simulink library "sm_trackV_lib_chain_underc_i1u2l7"  (R2026a)
settings: Solver=VariableStepAuto
undefined symbols (not defined in the file): Excv, Left, P1, P2, P3, P4, P5, P6, P7, P8, P9, Right
libraries: sm_trackV_lib_chain_underc_elem x26, sm_lib x24, nesl_utility x20, fl_lib x4, sm_trackV_lib_frame_i1u2l7 x2
(part 1 of 2)
Description:
  | Copyright 2023-2026 The MathWorks, Inc.
settings Model: Creator=smiller  LastModifiedBy=smiller

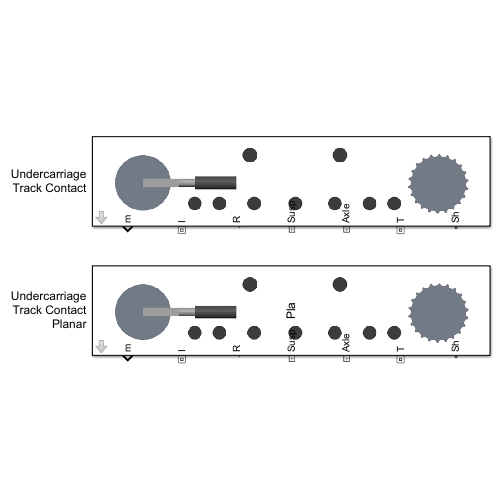
[thumbnail: Simulink's stored preview of the top-level diagram]
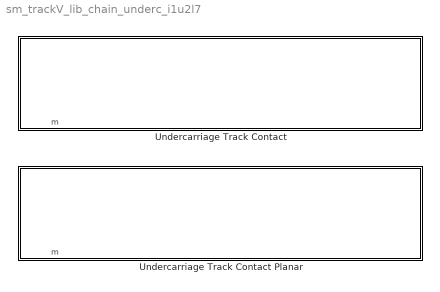
== system sm_trackV_lib_chain_underc_i1u2l7 ==
  Undercarriage Track Contact : Subsystem  mask(Undercarriage for Integration with Track Model){popup_leftOrRight=Left, sprk_xc=Excv.Sprocket.sprocket_xc, sprk_len=Excv.Sprocket.sprk_width, sprk_rho=Excv.Sprocket.density, sprk_clr=Excv.Sprocket.clr, sprk_opc=Excv.Sprocket.opc, sprk_contact_geo_ptcld=Excv.Sprocket.teeth_contact.ptcld.pts, sprk_contact_geo_rad=Excv.Sprocket.teeth_contact.ptcld.rad, sprk_contact_geo_clr=Excv.Sprocket.teeth_contact.ptcld.clr, sprk_contact_geo_opc=Excv.Sprocket.teeth_contact.ptcld.opc, idler_rad=Excv.Idler.rad, idler_len=Excv.Idler.len, idler_rho=Excv.Idler.rho, idler_clr=Excv.Idler.clr, idler_opc=Excv.Idler.opc, idler_contgeo_clr=Excv.Idler.chain_contact.clr, idler_contgeo_opc=Excv.Idler.chain_contact.opc, roller_upper_rad=Excv.Roller.Upper.rad, roller_upper_len=Excv.Roller.Upper.len, roller_upper_rho=Excv.Roller.Upper.rho, roller_upper_clr=Excv.Roller.Upper.clr, roller_upper_opc=Excv.Roller.Upper.opc, roller_upper_contgeo_clr=[1.0 0.0 0.0], roller_upper_contgeo_opc=1, roller_lower_rad=Excv.Roller.Lower.rad, roller_lower_len=Excv.Roller.Lower.len, roller_lower_rho=Excv.Roller.Lower.rho, roller_lower_clr=Excv.Roller.Lower.clr, roller_lower_opc=Excv.Roller.Lower.opc, roller_lower_contgeo_clr=[1.0 0.0 0.0], roller_lower_contgeo_opc=1, tensioner_cyl_len=Excv.Idler.Tensioner.cyl.len, tensioner_cyl_rad=Excv.Idler.Tensioner.cyl.rad, tensioner_cyl_rho=Excv.Idler.Tensioner.cyl.rho, tensioner_cyl_clr=Excv.Idler.Tensioner.cyl.clr, tensioner_cyl_opc=Excv.Idler.Tensioner.cyl.opc, tensioner_pist_len=Excv.Idler.Tensioner.piston.len, tensioner_pist_rad=Excv.Idler.Tensioner.piston.rad, tensioner_pist_rho=Excv.Idler.Tensioner.piston.rho, tensioner_pist_clr=Excv.Idler.Tensioner.piston.clr, tensioner_pist_opc=Excv.Idler.Tensioner.piston.opc, tensioner_br_length=Excv.Idler.Tensioner.bracket.len, tensioner_br_width=Excv.Idler.Tensioner.bracket.wid, tensioner_br_height=Excv.Idler.Tensioner.bracket.height, tensioner_br_thk=Excv.Idler.Tensioner.bracket.thk, tensioner_br_rho=Excv.Idler.Tensioner.bracket.rho, tensioner_br_clr=Excv.Idler.Tensioner.bracket.clr, tensioner_br_opc=Excv.Idler.Tensioner.bracket.opc, tensioner_eqpos=Excv.Idler.Tensioner.xeq, tensioner_x0=Excv.Idler.Tensioner.x0, tensioner_k=Excv.Idler.Tensioner.K, tensioner_b=Excv.Idler.Tensioner.B, roller_upper_x=Excv.Frame.Sprk2UpperX, roller_lower_x=Excv.Frame.Sprk2LowerX, idler_x=Excv.Frame.IdlerAssyX, axle_x=Excv.Frame.AxleX, roller_upper_y=Excv.Frame.Sprk2UpperY, roller_lower_y=Excv.Frame.Sprk2LowerY, idler_y=Excv.Frame.Sprk2IdlerY, axle_y=Excv.Frame.AxleY, frame_cg_offset=Excv.Frame.CGOffset, frame_mass=Excv.Frame.Mass, frame_moi=Excv.Frame.MOI, frame_poi=Excv.Frame.POI, frame_susp_offset=Excv.Frame.SuspOffset, popup_sense_roller=Actuator Torque}
      mask prompts: popup_leftOrRight "Left or Right"; sprk_xc "Extrusion Data [x y] (m)"; sprk_len "Length (m)"; sprk_rho "Density (kg/m^3)"; sprk_clr "Color [R G B] (0-1)"; sprk_opc "Opacity (0-1)"; sprk_contact_geo_ptcld "Point Cloud Data [x y z] (m)"; sprk_contact_geo_rad "Radius (m)"; sprk_contact_geo_clr "Color [R G B] (0-1)"; sprk_contact_geo_opc "Opacity (0-1)"; idler_rad "Radius (m)"; idler_len "Length (m)"; idler_rho "Density (kg/m^3)"; idler_clr "Color [R G B] (0-1)"; idler_opc "Opacity (0-1)"; idler_contgeo_clr "Color [R G B] (0-1)"; idler_contgeo_opc "Opacity (0-1)"; roller_upper_rad "Radius (m)"; roller_upper_len "Length (m)"; roller_upper_rho "Density (kg/m^3)"; roller_upper_clr "Color [R G B] (0-1)"; roller_upper_opc "Opacity (0-1)"; roller_upper_contgeo_clr "Color [R G B] (0-1)"; roller_upper_contgeo_opc "Opacity (0-1)"; roller_lower_rad "Radius (m)"; roller_lower_len "Length (m)"; roller_lower_rho "Density (kg/m^3)"; roller_lower_clr "Color [R G B] (0-1)"; roller_lower_opc "Opacity (0-1)"; roller_lower_contgeo_clr "Color [R G B] (0-1)"; roller_lower_contgeo_opc "Opacity (0-1)"; tensioner_cyl_len "Length (m)"; tensioner_cyl_rad "Radius (m)"; tensioner_cyl_rho "Density (kg/m^3)"; tensioner_cyl_clr "Color [R G B] (0-1)"; tensioner_cyl_opc "Opacity (0-1)"; tensioner_pist_len "Length (m)"; tensioner_pist_rad "Radius (m)"; tensioner_pist_rho "Density (kg/m^3)"; tensioner_pist_clr "Color [R G B] (0-1)"; tensioner_pist_opc "Opacity (0.1)"; tensioner_br_length "Length (m)"; tensioner_br_width "Width (m)"; tensioner_br_height "Height (m)"; tensioner_br_thk "Thickness (m)"; tensioner_br_rho "Density (kg/m^3)"; tensioner_br_clr "Color [R G B] (0-1)"; tensioner_br_opc "Opacity (0.1)"; tensioner_eqpos "Equilibrium Position (m)"; tensioner_x0 "Assembly Position (m)"; tensioner_k "Stiffness Coefficient (N/m)"; tensioner_b "Damping Coefficient (N/(m/s))"; roller_upper_x "Upper Rollers (vector) (m)"; roller_lower_x "Lower Rollers (vector) (m)"; idler_x "Idler Wheel (m)"; axle_x "Axle (m)"; roller_upper_y "Sprocket to Upper Rollers (m)"; roller_lower_y "Sprocket to Lower Rollers (m)"; idler_y "Sprocket to Idler (m)"; axle_y "Axle (m)"; frame_cg_offset "CG Offset from Sprocket [x y z] (m)"; frame_mass "Mass (kg)"; frame_moi "Moments of Inertia [Ixx Iyy Izz] (kg*m^2)"; frame_poi "Products of Inertia [Ixx Iyy Izz] (kg*m^2)"; frame_susp_offset "Suspension Offset from Sprocket [x y z] (m)"; popup_sense_roller "Roller"
      mask help: Models sprocket, rollers, and idler with tensioner. Components have contact geometry for integration with a segmented track model. The sprocket has a 1D rotational mechanical interface to the drivetrain.
      mask init:
      | bh = gcb;
      | set_param([bh '/Rollers'],'popup_sense_roller',get_param(bh,'popup_sense_roller'));
      mask TypeOptions popup_leftOrRight: Frame/popup_leftOrRight
      mask TypeOptions sprk_xc: Rollers/sprk_xc
      mask TypeOptions sprk_len: Rollers/sprk_len
      mask TypeOptions sprk_rho: Rollers/sprk_rho
      mask TypeOptions sprk_clr: Rollers/sprk_clr
      mask TypeOptions sprk_opc: Rollers/sprk_opc
      mask TypeOptions sprk_contact_geo_ptcld: Rollers/sprk_contact_geo_ptcld
      mask TypeOptions sprk_contact_geo_rad: Rollers/sprk_contact_geo_rad
      mask TypeOptions sprk_contact_geo_clr: Rollers/sprk_contact_geo_clr
      mask TypeOptions sprk_contact_geo_opc: Rollers/sprk_contact_geo_opc
      mask TypeOptions idler_rad: Rollers/idler_rad
      mask TypeOptions idler_len: Rollers/idler_len
      mask TypeOptions idler_rho: Rollers/idler_rho
      mask TypeOptions idler_clr: Rollers/idler_clr
      mask TypeOptions idler_opc: Rollers/idler_opc
      mask TypeOptions idler_contgeo_clr: Rollers/idler_contgeo_clr
      mask TypeOptions idler_contgeo_opc: Rollers/idler_contgeo_opc
      mask TypeOptions roller_upper_rad: Rollers/roller_upper_rad
      mask TypeOptions roller_upper_len: Rollers/roller_upper_len
      mask TypeOptions roller_upper_rho: Rollers/roller_upper_rho
      mask TypeOptions roller_upper_clr: Rollers/roller_upper_clr
      mask TypeOptions roller_upper_opc: Rollers/roller_upper_opc
      mask TypeOptions roller_upper_contgeo_clr: Rollers/roller_upper_contgeo_clr
      mask TypeOptions roller_upper_contgeo_opc: Rollers/roller_upper_contgeo_opc
      mask TypeOptions roller_lower_rad: Rollers/roller_lower_rad
      mask TypeOptions roller_lower_len: Rollers/roller_lower_len
      mask TypeOptions roller_lower_rho: Rollers/roller_lower_rho
      mask TypeOptions roller_lower_clr: Rollers/roller_lower_clr
      mask TypeOptions roller_lower_opc: Rollers/roller_lower_opc
      mask TypeOptions roller_lower_contgeo_clr: Rollers/roller_lower_contgeo_clr
      mask TypeOptions roller_lower_contgeo_opc: Rollers/roller_lower_contgeo_opc
      mask TypeOptions tensioner_cyl_len: Rollers/tensioner_cyl_len
      mask TypeOptions tensioner_cyl_rad: Rollers/tensioner_cyl_rad
      mask TypeOptions tensioner_cyl_rho: Rollers/tensioner_cyl_rho
      mask TypeOptions tensioner_cyl_clr: Rollers/tensioner_cyl_clr
      mask TypeOptions tensioner_cyl_opc: Rollers/tensioner_cyl_opc
      mask TypeOptions tensioner_pist_len: Rollers/tensioner_pist_len
      mask TypeOptions tensioner_pist_rad: Rollers/tensioner_pist_rad
      mask TypeOptions tensioner_pist_rho: Rollers/tensioner_pist_rho
      mask TypeOptions tensioner_pist_clr: Rollers/tensioner_pist_clr
      mask TypeOptions tensioner_pist_opc: Rollers/tensioner_pist_opc
      mask TypeOptions tensioner_br_length: Rollers/tensioner_br_length
      mask TypeOptions tensioner_br_width: Rollers/tensioner_br_width
      mask TypeOptions tensioner_br_height: Rollers/tensioner_br_height
      mask TypeOptions tensioner_br_thk: Rollers/tensioner_br_thk
      mask TypeOptions tensioner_br_rho: Rollers/tensioner_br_rho
      mask TypeOptions tensioner_br_clr: Rollers/tensioner_br_clr
      mask TypeOptions tensioner_br_opc: Rollers/tensioner_br_opc
      mask TypeOptions tensioner_eqpos: Rollers/tensioner_eqpos
      mask TypeOptions tensioner_x0: Rollers/tensioner_x0
      mask TypeOptions tensioner_k: Rollers/tensioner_k
      mask TypeOptions tensioner_b: Rollers/tensioner_b
      mask TypeOptions roller_upper_x: Frame/roller_upper_x
      mask TypeOptions roller_lower_x: Frame/roller_lower_x
      mask TypeOptions idler_x: Frame/idler_x
      mask TypeOptions axle_x: Frame/axle_x
      mask TypeOptions roller_upper_y: Frame/roller_upper_y
      mask TypeOptions roller_lower_y: Frame/roller_lower_y
      mask TypeOptions idler_y: Frame/idler_y
      mask TypeOptions axle_y: Frame/axle_y
      mask TypeOptions frame_cg_offset: Frame/frame_cg_offset
      mask TypeOptions frame_mass: Frame/frame_mass
      mask TypeOptions frame_moi: Frame/frame_moi
      mask TypeOptions frame_poi: Frame/frame_poi
      mask TypeOptions frame_susp_offset: Frame/frame_susp_offset
      mask TypeOptions popup_sense_roller: Constraint Force | Actuator Torque
      mask DialogControl cont_sprocket Prompt: Sprocket
      mask DialogControl cont_sprocket_solid Prompt: Solid
      mask DialogControl cont_sprocket_contact_geo Prompt: Contact Geometry
      mask DialogControl cont_idler Prompt: Idler
      mask DialogControl cont_idler_solid Prompt: Solid
      mask DialogControl cont_idler_contact_geo Prompt: Contact Geometry
      mask DialogControl cont_rollers Prompt: Rollers
      mask DialogControl cont_roller_upper Prompt: Upper
      mask DialogControl cont_roller_upper_contact_geo Prompt: Contact Geometry
      mask DialogControl cont_rollers_lower Prompt: Lower
      mask DialogControl cont_rollers_lower_contact_geo Prompt: Contact Geometry
      mask DialogControl cont_tensioner Prompt: Tensioner
      mask DialogControl cont_tensioner_cyl Prompt: Cylinder
      mask DialogControl cont_tensioner_pist Prompt: Piston
      mask DialogControl cont_tensioner_brkt Prompt: Bracket
      mask DialogControl cont_tensioner_assembly Prompt: Assembly
      mask DialogControl cont_frame Prompt: Frame
      mask DialogControl cont_offset_x Prompt: Longitudinal Offsets from Sprocket
      mask DialogControl cont_offset_y Prompt: Vertical Offsets
      mask DialogControl cont_mass Prompt: Mass and Inertia
      mask DialogControl cont_susp Prompt: Suspension Offsets
      mask DialogControl cont_sensing Prompt: Sensing
      mask Display: image('sm_excv_track_rollers_IMAGE.png');
  Undercarriage Track Contact Planar : Subsystem  mask(Undercarriage for Integration with Track Model){popup_leftOrRight=Right, sprk_xc=Excv.Sprocket.sprocket_xc, sprk_len=Excv.Sprocket.sprk_width, sprk_rho=Excv.Sprocket.density, sprk_clr=Excv.Sprocket.clr, sprk_opc=Excv.Sprocket.opc, sprk_contact_geo_ptcld=Excv.Sprocket.teeth_contact.ptcld.pts, sprk_contact_geo_rad=Excv.Sprocket.teeth_contact.ptcld.rad, sprk_contact_geo_clr=Excv.Sprocket.teeth_contact.ptcld.clr, sprk_contact_geo_opc=Excv.Sprocket.teeth_contact.ptcld.opc, idler_rad=Excv.Idler.rad, idler_len=Excv.Idler.len, idler_rho=Excv.Idler.rho, idler_clr=Excv.Idler.clr, idler_opc=Excv.Idler.opc, idler_contgeo_clr=Excv.Idler.chain_contact.clr, idler_contgeo_opc=Excv.Idler.chain_contact.opc, roller_upper_rad=Excv.Roller.Upper.rad, roller_upper_len=Excv.Roller.Upper.len, roller_upper_rho=Excv.Roller.Upper.rho, roller_upper_clr=Excv.Roller.Upper.clr, roller_upper_opc=Excv.Roller.Upper.opc, roller_upper_contgeo_clr=[1.0 0.0 0.0], roller_upper_contgeo_opc=1, roller_lower_rad=Excv.Roller.Lower.rad, roller_lower_len=Excv.Roller.Lower.len, roller_lower_rho=Excv.Roller.Lower.rho, roller_lower_clr=Excv.Roller.Lower.clr, roller_lower_opc=Excv.Roller.Lower.opc, roller_lower_contgeo_clr=[1.0 0.0 0.0], roller_lower_contgeo_opc=1, tensioner_cyl_len=Excv.Idler.Tensioner.cyl.len, tensioner_cyl_rad=Excv.Idler.Tensioner.cyl.rad, tensioner_cyl_rho=Excv.Idler.Tensioner.cyl.rho, tensioner_cyl_clr=Excv.Idler.Tensioner.cyl.clr, tensioner_cyl_opc=Excv.Idler.Tensioner.cyl.opc, tensioner_pist_len=Excv.Idler.Tensioner.piston.len, tensioner_pist_rad=Excv.Idler.Tensioner.piston.rad, tensioner_pist_rho=Excv.Idler.Tensioner.piston.rho, tensioner_pist_clr=Excv.Idler.Tensioner.piston.clr, tensioner_pist_opc=Excv.Idler.Tensioner.piston.opc, tensioner_br_length=Excv.Idler.Tensioner.bracket.len, tensioner_br_width=Excv.Idler.Tensioner.bracket.wid, tensioner_br_height=Excv.Idler.Tensioner.bracket.height, tensioner_br_thk=Excv.Idler.Tensioner.bracket.thk, tensioner_br_rho=Excv.Idler.Tensioner.bracket.rho, tensioner_br_clr=Excv.Idler.Tensioner.bracket.clr, tensioner_br_opc=Excv.Idler.Tensioner.bracket.opc, tensioner_eqpos=Excv.Idler.Tensioner.xeq, tensioner_x0=Excv.Idler.Tensioner.x0, tensioner_k=Excv.Idler.Tensioner.K, tensioner_b=Excv.Idler.Tensioner.B, roller_upper_x=Excv.Frame.Sprk2UpperX, roller_lower_x=Excv.Frame.Sprk2LowerX, idler_x=Excv.Frame.IdlerAssyX, axle_x=Excv.Frame.AxleX, roller_upper_y=Excv.Frame.Sprk2UpperY, roller_lower_y=Excv.Frame.Sprk2LowerY, idler_y=Excv.Frame.Sprk2IdlerY, axle_y=Excv.Frame.AxleY, frame_cg_offset=Excv.Frame.CGOffset, frame_mass=Excv.Frame.Mass, frame_moi=Excv.Frame.MOI, frame_poi=Excv.Frame.POI, frame_susp_offset=Excv.Frame.SuspOffset, popup_sense_roller=Actuator Torque}
      mask prompts: popup_leftOrRight "Left or Right"; sprk_xc "Extrusion Data [x y] (m)"; sprk_len "Length (m)"; sprk_rho "Density (kg/m^3)"; sprk_clr "Color [R G B] (0-1)"; sprk_opc "Opacity (0-1)"; sprk_contact_geo_ptcld "Point Cloud Data [x y z] (m)"; sprk_contact_geo_rad "Radius (m)"; sprk_contact_geo_clr "Color [R G B] (0-1)"; sprk_contact_geo_opc "Opacity (0-1)"; idler_rad "Radius (m)"; idler_len "Length (m)"; idler_rho "Density (kg/m^3)"; idler_clr "Color [R G B] (0-1)"; idler_opc "Opacity (0-1)"; idler_contgeo_clr "Color [R G B] (0-1)"; idler_contgeo_opc "Opacity (0-1)"; roller_upper_rad "Radius (m)"; roller_upper_len "Length (m)"; roller_upper_rho "Density (kg/m^3)"; roller_upper_clr "Color [R G B] (0-1)"; roller_upper_opc "Opacity (0-1)"; roller_upper_contgeo_clr "Color [R G B] (0-1)"; roller_upper_contgeo_opc "Opacity (0-1)"; roller_lower_rad "Radius (m)"; roller_lower_len "Length (m)"; roller_lower_rho "Density (kg/m^3)"; roller_lower_clr "Color [R G B] (0-1)"; roller_lower_opc "Opacity (0-1)"; roller_lower_contgeo_clr "Color [R G B] (0-1)"; roller_lower_contgeo_opc "Opacity (0-1)"; tensioner_cyl_len "Length (m)"; tensioner_cyl_rad "Radius (m)"; tensioner_cyl_rho "Density (kg/m^3)"; tensioner_cyl_clr "Color [R G B] (0-1)"; tensioner_cyl_opc "Opacity (0-1)"; tensioner_pist_len "Length (m)"; tensioner_pist_rad "Radius (m)"; tensioner_pist_rho "Density (kg/m^3)"; tensioner_pist_clr "Color [R G B] (0-1)"; tensioner_pist_opc "Opacity (0.1)"; tensioner_br_length "Length (m)"; tensioner_br_width "Width (m)"; tensioner_br_height "Height (m)"; tensioner_br_thk "Thickness (m)"; tensioner_br_rho "Density (kg/m^3)"; tensioner_br_clr "Color [R G B] (0-1)"; tensioner_br_opc "Opacity (0.1)"; tensioner_eqpos "Equilibrium Position (m)"; tensioner_x0 "Assembly Position (m)"; tensioner_k "Stiffness Coefficient (N/m)"; tensioner_b "Damping Coefficient (N/(m/s))"; roller_upper_x "Upper Rollers (vector) (m)"; roller_lower_x "Lower Rollers (vector) (m)"; idler_x "Idler Wheel (m)"; axle_x "Axle (m)"; roller_upper_y "Sprocket to Upper Rollers (m)"; roller_lower_y "Sprocket to Lower Rollers (m)"; idler_y "Sprocket to Idler (m)"; axle_y "Sprocket to Axle (m)"; frame_cg_offset "CG Offset from Sprocket [x y z] (m)"; frame_mass "Mass (kg)"; frame_moi "Moments of Inertia [Ixx Iyy Izz] (kg*m^2)"; frame_poi "Products of Inertia [Ixx Iyy Izz] (kg*m^2)"; frame_susp_offset "Suspension Offset from Sprocket [x y z] (m)"; popup_sense_roller "Roller"
      mask help: Models sprocket, rollers, and idler with tensioner. Components have contact geometry for integration with a segmented track model. Contact forces within the track are planar to speed up simulation. The sprocket has a 1D rotational mechanical interface to the drivetrain.
      mask init:
      | bh = gcb;
      | set_param([bh '/Rollers'],'popup_sense_roller',get_param(bh,'popup_sense_roller'));
      mask TypeOptions popup_leftOrRight: Frame/popup_leftOrRight
      mask TypeOptions sprk_xc: Rollers/sprk_xc
      mask TypeOptions sprk_len: Rollers/sprk_len
      mask TypeOptions sprk_rho: Rollers/sprk_rho
      mask TypeOptions sprk_clr: Rollers/sprk_clr
      mask TypeOptions sprk_opc: Rollers/sprk_opc
      mask TypeOptions sprk_contact_geo_ptcld: Rollers/sprk_contact_geo_ptcld
      mask TypeOptions sprk_contact_geo_rad: Rollers/sprk_contact_geo_rad
      mask TypeOptions sprk_contact_geo_clr: Rollers/sprk_contact_geo_clr
      mask TypeOptions sprk_contact_geo_opc: Rollers/sprk_contact_geo_opc
      mask TypeOptions idler_rad: Rollers/idler_rad
      mask TypeOptions idler_len: Rollers/idler_len
      mask TypeOptions idler_rho: Rollers/idler_rho
      mask TypeOptions idler_clr: Rollers/idler_clr
      mask TypeOptions idler_opc: Rollers/idler_opc
      mask TypeOptions idler_contgeo_clr: Rollers/idler_contgeo_clr
      mask TypeOptions idler_contgeo_opc: Rollers/idler_contgeo_opc
      mask TypeOptions roller_upper_rad: Rollers/roller_upper_rad
      mask TypeOptions roller_upper_len: Rollers/roller_upper_len
      mask TypeOptions roller_upper_rho: Rollers/roller_upper_rho
      mask TypeOptions roller_upper_clr: Rollers/roller_upper_clr
      mask TypeOptions roller_upper_opc: Rollers/roller_upper_opc
      mask TypeOptions roller_upper_contgeo_clr: Rollers/roller_upper_contgeo_clr
      mask TypeOptions roller_upper_contgeo_opc: Rollers/roller_upper_contgeo_opc
      mask TypeOptions roller_lower_rad: Rollers/roller_lower_rad
      mask TypeOptions roller_lower_len: Rollers/roller_lower_len
      mask TypeOptions roller_lower_rho: Rollers/roller_lower_rho
      mask TypeOptions roller_lower_clr: Rollers/roller_lower_clr
      mask TypeOptions roller_lower_opc: Rollers/roller_lower_opc
      mask TypeOptions roller_lower_contgeo_clr: Rollers/roller_lower_contgeo_clr
      mask TypeOptions roller_lower_contgeo_opc: Rollers/roller_lower_contgeo_opc
      mask TypeOptions tensioner_cyl_len: Rollers/tensioner_cyl_len
      mask TypeOptions tensioner_cyl_rad: Rollers/tensioner_cyl_rad
      mask TypeOptions tensioner_cyl_rho: Rollers/tensioner_cyl_rho
      mask TypeOptions tensioner_cyl_clr: Rollers/tensioner_cyl_clr
      mask TypeOptions tensioner_cyl_opc: Rollers/tensioner_cyl_opc
      mask TypeOptions tensioner_pist_len: Rollers/tensioner_pist_len
      mask TypeOptions tensioner_pist_rad: Rollers/tensioner_pist_rad
      mask TypeOptions tensioner_pist_rho: Rollers/tensioner_pist_rho
      mask TypeOptions tensioner_pist_clr: Rollers/tensioner_pist_clr
      mask TypeOptions tensioner_pist_opc: Rollers/tensioner_pist_opc
      mask TypeOptions tensioner_br_length: Rollers/tensioner_br_length
      mask TypeOptions tensioner_br_width: Rollers/tensioner_br_width
      mask TypeOptions tensioner_br_height: Rollers/tensioner_br_height
      mask TypeOptions tensioner_br_thk: Rollers/tensioner_br_thk
      mask TypeOptions tensioner_br_rho: Rollers/tensioner_br_rho
      mask TypeOptions tensioner_br_clr: Rollers/tensioner_br_clr
      mask TypeOptions tensioner_br_opc: Rollers/tensioner_br_opc
      mask TypeOptions tensioner_eqpos: Rollers/tensioner_eqpos
      mask TypeOptions tensioner_x0: Rollers/tensioner_x0
      mask TypeOptions tensioner_k: Rollers/tensioner_k
      mask TypeOptions tensioner_b: Rollers/tensioner_b
      mask TypeOptions roller_upper_x: Frame/roller_upper_x
      mask TypeOptions roller_lower_x: Frame/roller_lower_x
      mask TypeOptions idler_x: Frame/idler_x
      mask TypeOptions axle_x: Frame/axle_x
      mask TypeOptions roller_upper_y: Frame/roller_upper_y
      mask TypeOptions roller_lower_y: Frame/roller_lower_y
      mask TypeOptions idler_y: Frame/idler_y
      mask TypeOptions axle_y: Frame/axle_y
      mask TypeOptions frame_cg_offset: Frame/frame_cg_offset
      mask TypeOptions frame_mass: Frame/frame_mass
      mask TypeOptions frame_moi: Frame/frame_moi
      mask TypeOptions frame_poi: Frame/frame_poi
      mask TypeOptions frame_susp_offset: Frame/frame_susp_offset
      mask TypeOptions popup_sense_roller: Constraint Force | Actuator Torque
      mask DialogControl cont_sprocket Prompt: Sprocket
      mask DialogControl cont_sprocket_solid Prompt: Solid
      mask DialogControl cont_sprocket_contact_geo Prompt: Contact Geometry
      mask DialogControl cont_idler Prompt: Idler
      mask DialogControl cont_idler_solid Prompt: Solid
      mask DialogControl cont_idler_contact_geo Prompt: Contact Geometry
      mask DialogControl cont_rollers Prompt: Rollers
      mask DialogControl cont_roller_upper Prompt: Upper
      mask DialogControl cont_roller_upper_contact_geo Prompt: Contact Geometry
      mask DialogControl cont_rollers_lower Prompt: Lower
      mask DialogControl cont_rollers_lower_contact_geo Prompt: Contact Geometry
      mask DialogControl cont_tensioner Prompt: Tensioner
      mask DialogControl cont_tensioner_cyl Prompt: Cylinder
      mask DialogControl cont_tensioner_pist Prompt: Piston
      mask DialogControl cont_tensioner_brkt Prompt: Bracket
      mask DialogControl cont_tensioner_assembly Prompt: Assembly
      mask DialogControl cont_frame Prompt: Frame
      mask DialogControl cont_offset_x Prompt: Longitudinal Offsets from Sprocket
      mask DialogControl cont_offset_y Prompt: Vertical Offsets
      mask DialogControl cont_mass Prompt: Mass and Inertia
      mask DialogControl cont_susp Prompt: Suspension Offset
      mask DialogControl cont_sensing Prompt: Sensing
      mask Display:
      | image('sm_excv_track_rollers_IMAGE.png');
      | disp('Pla');

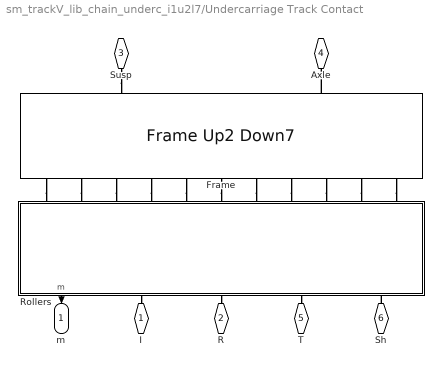
== system sm_trackV_lib_chain_underc_i1u2l7/Undercarriage Track Contact ==
  Frame : sm_trackV_lib_frame_i1u2l7/Frame Up2 Down7  popup_leftOrRight=Left  roller_upper_x=roller_upper_x  roller_lower_x=roller_lower_x  idler_x=idler_x  axle_x=axle_x  roller_upper_y=roller_upper_y  roller_lower_y=roller_lower_y  idler_y=idler_y  axle_y=axle_y  frame_cg_offset=frame_cg_offset  frame_mass=frame_mass  frame_moi=frame_moi  frame_poi=frame_poi  frame_susp_offset=frame_susp_offset
  Rollers : Subsystem  mask(Rollers for Integration with Track Model){sprk_xc=sprk_xc, sprk_len=sprk_len, sprk_rho=sprk_rho, sprk_clr=sprk_clr, sprk_opc=sprk_opc, sprk_contact_geo_ptcld=sprk_contact_geo_ptcld, sprk_contact_geo_rad=sprk_contact_geo_rad, sprk_contact_geo_clr=sprk_contact_geo_clr, sprk_contact_geo_opc=sprk_contact_geo_opc, idler_rad=idler_rad, idler_len=idler_len, idler_rho=idler_rho, idler_clr=idler_clr, idler_opc=idler_opc, idler_contgeo_clr=idler_contgeo_clr, idler_contgeo_opc=idler_contgeo_opc, roller_upper_len=roller_upper_len, roller_upper_rad=roller_upper_rad, roller_upper_rho=roller_upper_rho, roller_upper_clr=roller_upper_clr, roller_upper_opc=roller_upper_opc, roller_upper_contgeo_clr=roller_upper_contgeo_clr, roller_upper_contgeo_opc=roller_upper_contgeo_opc, roller_lower_len=roller_lower_len, roller_lower_rad=roller_lower_rad, roller_lower_rho=roller_lower_rho, roller_lower_clr=roller_lower_clr, roller_lower_opc=roller_lower_opc, roller_lower_contgeo_clr=roller_lower_contgeo_clr, roller_lower_contgeo_opc=roller_lower_contgeo_opc, tensioner_cyl_rad=tensioner_cyl_rad, tensioner_cyl_len=tensioner_cyl_len, tensioner_cyl_rho=tensioner_cyl_rho, tensioner_cyl_clr=tensioner_cyl_clr, tensioner_cyl_opc=tensioner_cyl_opc, tensioner_pist_rad=tensioner_pist_rad, tensioner_pist_len=tensioner_pist_len, tensioner_pist_rho=tensioner_pist_rho, tensioner_pist_clr=tensioner_pist_clr, tensioner_pist_opc=tensioner_pist_opc, tensioner_br_length=tensioner_br_length, tensioner_br_width=tensioner_br_width, tensioner_br_height=tensioner_br_height, tensioner_br_thk=tensioner_br_thk, tensioner_br_rho=tensioner_br_rho, tensioner_br_clr=tensioner_br_clr, tensioner_br_opc=tensioner_br_opc, tensioner_eqpos=tensioner_eqpos, tensioner_x0=tensioner_x0, tensioner_b=tensioner_b, tensioner_k=tensioner_k, popup_sense_roller=Actuator Torque}
      mask prompts: sprk_xc "Extrusion Data [x y] (m)"; sprk_len "Length (m)"; sprk_rho "Density (kg/m^3)"; sprk_clr "Color [R G B] (0-1)"; sprk_opc "Opacity (0-1)"; sprk_contact_geo_ptcld "Point Cloud Data [x y z] (m)"; sprk_contact_geo_rad "Radius (m)"; sprk_contact_geo_clr "Color [R G B] (0-1)"; sprk_contact_geo_opc "Opacity (0-1)"; idler_rad "Radius (m)"; idler_len "Length(m)"; idler_rho "Density (kg/m^3)"; idler_clr "Color [R G B] (0-1)"; idler_opc "Opacity (0-1)"; idler_contgeo_clr "Color [R G B] (0-1)"; idler_contgeo_opc "Opacity (0-1)"; roller_upper_len "Length (m)"; roller_upper_rad "Radius (m)"; roller_upper_rho "Density (kg/m^3)"; roller_upper_clr "Color [R G B] (0-1)"; roller_upper_opc "Opacity (0-1)"; roller_upper_contgeo_clr "Color [R G B] (0-1)"; roller_upper_contgeo_opc "Opacity (0-1)"; roller_lower_len "Length (m)"; roller_lower_rad "Radius (m)"; roller_lower_rho "Density (kg/m^3)"; roller_lower_clr "Color [R G B] (0-1)"; roller_lower_opc "Opacity (0-1)"; roller_lower_contgeo_clr "Color [R G B] (0-1)"; roller_lower_contgeo_opc "Opacity (0-1)"; tensioner_cyl_rad "Radius (m)"; tensioner_cyl_len "Length (m)"; tensioner_cyl_rho "Density (kg/m^3)"; tensioner_cyl_clr "Color [R G B] (0-1)"; tensioner_cyl_opc "Opacity (0-1)"; tensioner_pist_rad "Radius (m)"; tensioner_pist_len "Length (m)"; tensioner_pist_rho "Density (kg/m^3)"; tensioner_pist_clr "Color [R G B] (0-1)"; tensioner_pist_opc "Opacity (0.1)"; tensioner_br_length "Length (m)"; tensioner_br_width "Width (m)"; tensioner_br_height "Height (m)"; tensioner_br_thk "Thickness (m)"; tensioner_br_rho "Density (kg/m^3)"; tensioner_br_clr "Color [R G B] (0-1)"; tensioner_br_opc "Opacity (0.1)"; tensioner_eqpos "Equilibrium Position (m)"; tensioner_x0 "Assembly Position (m)"; tensioner_b "Damping Coefficient (N/(m/s))"; tensioner_k "Stiffness Coefficient (N/m)"; popup_sense_roller "Roller"
      mask help: Models sprocket, rollers, and idler with tensioner. Components have contact geometry for integration with a segmented track model. The sprocket has a 1D rotational mechanical interface to the drivetrain.
      mask init:
      | % Sensing a constraint force can be computationally expensive
      | % Use popup to turn it off if quantity is not needed
      | bh = gcb;
      | if(strcmp(get_param(bh,'popup_sense_roller'),'Constraint Force'))
      |     SCF = 'on'; STF = 'off';
      |     connectedPort = "fc_out";
      |     senseConstraintTorque = "on";
      |     senseTorqueForce = "off";
      | 
      | else
      |     SCF = 'off'; STF = 'on';
      |     connectedPort = "t_out";
      |     senseConstraintTorque = "off";
      |     senseTorqueForce = "on";
      | end
      | 
      | f = Simulink.FindOptions('RegExp',true,'SearchDepth',1);
      | bh_rv = Simulink.findBlocks(bh,'Name','Revolute Lower #*',f);
      | bh_ps = Simulink.findBlocks(bh,'Name','PS-SL Lower #*',f);
      | [~, indrv] = sort(getfullname(bh_rv));
      | [~, indps] = sort(getfullname(bh_ps));
      | bh_rv = bh_rv(indrv);
      | bh_ps = bh_ps(indps);
      | 
      | bh_rvspr = get_param([bh '/Revolute Sprocket'],'Handle');
      | bh_rvidl = get_param([bh '/Revolute Idler'],'Handle');
      | 
      | bh_psspr = get_param([bh '/PS-SL Sprocket'],'Handle');
      | bh_psidl = get_param([bh '/PS-SL Idler'],'Handle');
      | 
      | bh_rv = [bh_rv; bh_rvidl; bh_rvspr];
      | bh_ps = [bh_ps; bh_psidl; bh_psspr];
      | 
      | for i = 1:length(bh_rv)
      |     port_rv = get_param(bh_rv(i),'PortHandles');
      |     port_ps = get_param(bh_ps(i),'PortHandles');
      |     line_rv = get_param(bh_rv(i),'LineHandles');
      | 
      |     if (i==length(bh_rv))
      |         lineInd = 3; % Sprocket joint senses 2 signals
      |     else
      |         lineInd = 2; % All other joints sense 1 signal
      |     end
      |     delete_line(line_rv.RConn(lineInd))
      | 
      |     set_param(bh_rv(i),'SenseConstraintForce',SCF,'SenseTorqueForce',STF);
      |     simscape.addConnection(bh_rv(i), connectedPort, bh_ps(i),'input');
      | 
      | end
      mask TypeOptions sprk_xc: Sprocket/sprk_xc
      mask TypeOptions sprk_len: Sprocket/sprk_len
      mask TypeOptions sprk_rho: Sprocket/sprk_rho
      mask TypeOptions sprk_clr: Sprocket/sprk_clr
      mask TypeOptions sprk_opc: Sprocket/sprk_opc
      mask TypeOptions sprk_contact_geo_ptcld: Sprocket/sprk_contact_geo_ptcld
      mask TypeOptions sprk_contact_geo_rad: Sprocket/sprk_contact_geo_rad
      mask TypeOptions sprk_contact_geo_clr: Sprocket/sprk_contact_geo_clr
      mask TypeOptions sprk_contact_geo_opc: Sprocket/sprk_contact_geo_opc
      mask TypeOptions idler_rad: Idler/idler_rad
      mask TypeOptions idler_len: Idler/idler_len
      mask TypeOptions idler_rho: Idler/idler_rho
      mask TypeOptions idler_clr: Idler/idler_clr
      mask TypeOptions idler_opc: Idler/idler_opc
      mask TypeOptions idler_contgeo_clr: Idler/idler_contgeo_clr
      mask TypeOptions idler_contgeo_opc: Idler/idler_contgeo_opc
      mask TypeOptions roller_upper_len:
      | Roller
      | Upper 1/roller_upper_len | Roller
      | Upper 2/roller_upper_len
      mask TypeOptions roller_upper_rad:
      | Roller
      | Upper 1/roller_upper_rad | Roller
      | Upper 2/roller_upper_rad
      mask TypeOptions roller_upper_rho:
      | Roller
      | Upper 1/roller_upper_rho | Roller
      | Upper 2/roller_upper_rho
      mask TypeOptions roller_upper_clr:
      | Roller
      | Upper 1/roller_upper_clr | Roller
      | Upper 2/roller_upper_clr
      mask TypeOptions roller_upper_opc:
      | Roller
      | Upper 1/roller_upper_opc | Roller
      | Upper 2/roller_upper_opc
      mask TypeOptions roller_upper_contgeo_clr:
      | Roller
      | Upper 1/roller_upper_contgeo_clr | Roller
      | Upper 2/roller_upper_contgeo_clr
      mask TypeOptions roller_upper_contgeo_opc:
      | Roller
      | Upper 1/roller_upper_contgeo_opc | Roller
      | Upper 2/roller_upper_contgeo_opc
      mask TypeOptions roller_lower_len:
      | Roller
      | Lower 1/roller_lower_len | Roller
      | Lower 2/roller_lower_len | Roller
      | Lower 3/roller_lower_len | Roller
      | Lower 4/roller_lower_len | Roller
      | Lower 5/roller_lower_len | Roller
      | Lower 6/roller_lower_len | Roller
      | Lower 7/roller_lower_len
      mask TypeOptions roller_lower_rad:
      | Roller
      | Lower 1/roller_lower_rad | Roller
      | Lower 2/roller_lower_rad | Roller
      | Lower 3/roller_lower_rad | Roller
      | Lower 4/roller_lower_rad | Roller
      | Lower 5/roller_lower_rad | Roller
      | Lower 6/roller_lower_rad | Roller
      | Lower 7/roller_lower_rad
      mask TypeOptions roller_lower_rho:
      | Roller
      | Lower 1/roller_lower_rho | Roller
      | Lower 2/roller_lower_rho | Roller
      | Lower 3/roller_lower_rho | Roller
      | Lower 4/roller_lower_rho | Roller
      | Lower 5/roller_lower_rho | Roller
      | Lower 6/roller_lower_rho | Roller
      | Lower 7/roller_lower_rho
      mask TypeOptions roller_lower_clr:
      | Roller
      | Lower 1/roller_lower_clr | Roller
      | Lower 2/roller_lower_clr | Roller
      | Lower 3/roller_lower_clr | Roller
      | Lower 4/roller_lower_clr | Roller
      | Lower 5/roller_lower_clr | Roller
      | Lower 6/roller_lower_clr | Roller
      | Lower 7/roller_lower_clr
      mask TypeOptions roller_lower_opc:
      | Roller
      | Lower 1/roller_lower_opc | Roller
      | Lower 2/roller_lower_opc | Roller
      | Lower 3/roller_lower_opc | Roller
      | Lower 4/roller_lower_opc | Roller
      | Lower 5/roller_lower_opc | Roller
      | Lower 6/roller_lower_opc | Roller
      | Lower 7/roller_lower_opc
      mask TypeOptions roller_lower_contgeo_clr:
      | Roller
      | Lower 1/roller_lower_contgeo_clr | Roller
      | Lower 2/roller_lower_contgeo_clr | Roller
      | Lower 3/roller_lower_contgeo_clr | Roller
      | Lower 4/roller_lower_contgeo_clr | Roller
      | Lower 5/roller_lower_contgeo_clr | Roller
      | Lower 6/roller_lower_contgeo_clr | Roller
      | Lower 7/roller_lower_contgeo_clr
      mask TypeOptions roller_lower_contgeo_opc:
      | Roller
      | Lower 1/roller_lower_contgeo_opc | Roller
      | Lower 2/roller_lower_contgeo_opc | Roller
      | Lower 3/roller_lower_contgeo_opc | Roller
      | Lower 4/roller_lower_contgeo_opc | Roller
      | Lower 5/roller_lower_contgeo_opc | Roller
      | Lower 6/roller_lower_contgeo_opc | Roller
      | Lower 7/roller_lower_contgeo_opc
      mask TypeOptions tensioner_cyl_rad:
      | Tensioner
      | Cylinder/cyl_rad
      mask TypeOptions tensioner_cyl_len:
      | Tensioner
      | Cylinder/cyl_len
      mask TypeOptions tensioner_cyl_rho:
      | Tensioner
      | Cylinder/cyl_rho
      mask TypeOptions tensioner_cyl_clr:
      | Tensioner
      | Cylinder/cyl_clr
      mask TypeOptions tensioner_cyl_opc:
      | Tensioner
      | Cylinder/cyl_opc
      mask TypeOptions tensioner_pist_rad:
      | Tensioner
      | Piston/pist_rad
      mask TypeOptions tensioner_pist_len:
      | Tensioner
      | Piston/pist_len
      mask TypeOptions tensioner_pist_rho:
      | Tensioner
      | Piston/pist_rho
      mask TypeOptions tensioner_pist_clr:
      | Tensioner
      | Piston/pist_clr
      mask TypeOptions tensioner_pist_opc:
      | Tensioner
      | Piston/pist_opc
      mask TypeOptions tensioner_br_length:
      | Tensioner
      | Piston/br_length
      mask TypeOptions tensioner_br_width:
      | Tensioner
      | Piston/br_width
      mask TypeOptions tensioner_br_height:
      | Tensioner
      | Piston/br_height
      mask TypeOptions tensioner_br_thk:
      | Tensioner
      | Piston/br_thk
      mask TypeOptions tensioner_br_rho:
      | Tensioner
      | Piston/br_rho
      mask TypeOptions tensioner_br_clr:
      | Tensioner
      | Piston/br_clr
      mask TypeOptions tensioner_br_opc:
      | Tensioner
      | Piston/br_opc
      mask TypeOptions tensioner_eqpos:
      | Prismatic
      | Tensioner/EquilibriumPosition
      mask TypeOptions tensioner_x0:
      | Prismatic
      | Tensioner/PositionTargetValue
      mask TypeOptions tensioner_b:
      | Prismatic
      | Tensioner/DampingCoefficient
      mask TypeOptions tensioner_k:
      | Prismatic
      | Tensioner/SpringStiffness
      mask TypeOptions popup_sense_roller: Constraint Force | Actuator Torque
      mask DialogControl cont_sprk Prompt: Sprocket
      mask DialogControl cont_sprk_solid Prompt: Solid
      mask DialogControl cont_sprk_contact_geo Prompt: Contact Geometry
      mask DialogControl cont_idler Prompt: Idler
      mask DialogControl cont_idler_solid Prompt: Solid
      mask DialogControl cont_idler_contact_geo Prompt: Contact Geometry
      mask DialogControl cont_rollers Prompt: Rollers
      mask DialogControl cont_roller_upper Prompt: Upper
      mask DialogControl cont_roller_upper_contact_geo Prompt: Contact Geometry
      mask DialogControl cont_lower Prompt: Lower
      mask DialogControl cont_lower_contact_geo Prompt: Contact Geometry
      mask DialogControl cont_tensioner Prompt: Tensioner
      mask DialogControl cont_tensioner_cyl Prompt: Cylinder
      mask DialogControl cont_tensioner_pist Prompt: Piston
      mask DialogControl cont_tensioner_brkt Prompt: Bracket
      mask DialogControl cont_tensioner_assy Prompt: Assembly
      mask DialogControl Container20 Prompt: Sensing
      mask Display: image('sm_excv_track_rollers_IMAGE.png');
  I : PMIOPort  Side=Right
  R : PMIOPort  Port=2  Side=Right
  Susp : PMIOPort  Port=3  Side=Right
  Axle : PMIOPort  Port=4  Side=Right
  T : PMIOPort  Port=5  Side=Right
  Sh : PMIOPort  Port=6  Side=Right
  m : Outport
  wires:
  Rollers/1(m) -> m/1
  connections:
  Susp/RConn1 -- Frame/LConn1
  Rollers/RConn2 -- R/RConn1
  Frame/LConn2 -- Axle/RConn1
  Rollers/RConn1 -- I/RConn1
  Rollers/RConn3 -- T/RConn1
  Frame/RConn7 -- Rollers/LConn7
  Frame/RConn5 -- Rollers/LConn5
  Frame/RConn4 -- Rollers/LConn4
  Frame/RConn8 -- Rollers/LConn8
  Frame/RConn10 -- Rollers/LConn10
  Frame/RConn9 -- Rollers/LConn9
  Frame/RConn6 -- Rollers/LConn6
  Frame/RConn1 -- Rollers/LConn1
  Frame/RConn11 -- Rollers/LConn11
  Frame/RConn3 -- Rollers/LConn3
  Frame/RConn2 -- Rollers/LConn2
  Sh/RConn1 -- Rollers/RConn4
